simulink model "V605_rotorModel"  (R2025a)
settings: Solver=FixedStepAuto  StartTime=0.0  StopTime=10.0  RelTol=1e-3
undefined symbols (not defined in the file or in its folder): motor
libraries: simulink x1
settings Model: Creator=Ayush_S  LastModifiedBy=Ayush_S

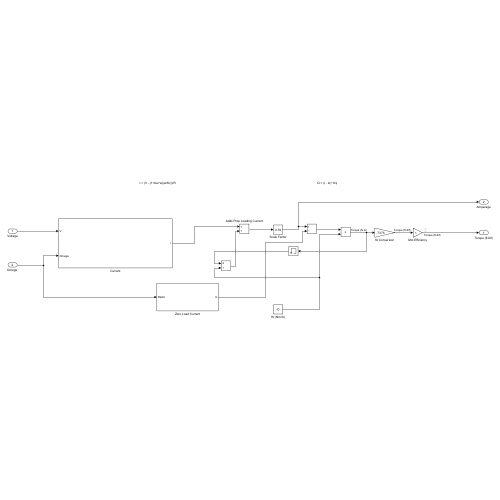
[thumbnail: Simulink's stored preview of the top-level diagram]
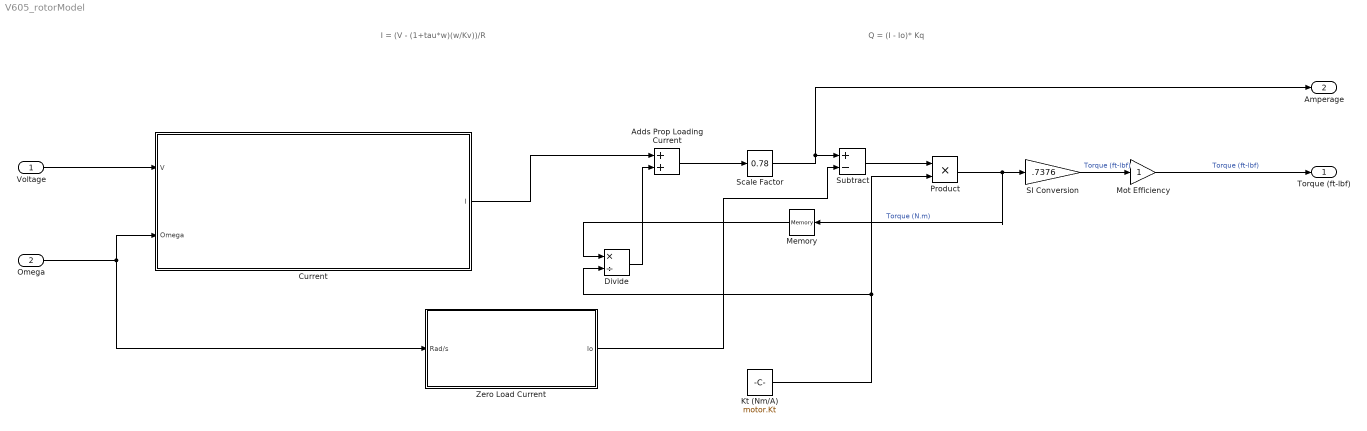
== system V605_rotorModel ==
  note: Q = (I - Io)* Kq
  note: I = (V - (1+tau*w)(w/Kv))/R
  Voltage : Inport
  "Omega " : Inport  Port=2
  Adds Prop Loading Current : Sum
  Current : Subsystem
  Divide : Product  Inputs=*/
  Kt (Nm/A) : Constant  Value=motor.Kt
  Memory : Memory
  Mot Efficiency : Gain
  Product : Product
  SI Conversion : Gain  Gain=.7376
  Scale Factor : simulink/Math Operations/Slider Gain  gain=0.78  low=0  high=2
  Subtract : Sum  Inputs=+-
  Zero Load Current : Subsystem
  Torque (ft-lbf) : Outport
  Amperage : Outport  Port=2
  wires:
  "Omega "/1 -> Current/2(Omega), Zero Load Current/1(Rad/s)
  Zero Load Current/1(Io) -> Subtract/2
  Scale Factor/1 -> Amperage/1, Subtract/1
  Divide/1 -> Adds Prop Loading Current/2
  Product/1 -> Memory/1, SI Conversion/1  "Torque (N.m)"
  Kt (Nm/A)/1 -> Divide/2, Product/2
  Mot Efficiency/1 -> Torque (ft-lbf)/1  "Torque (ft-lbf)"
  Subtract/1 -> Product/1
  Voltage/1 -> Current/1(V)
  Adds Prop Loading Current/1 -> Scale Factor/1
  SI Conversion/1 -> Mot Efficiency/1  "Torque (ft-lbf)"
  Current/1(I) -> Adds Prop Loading Current/1
  Memory/1 -> Divide/1

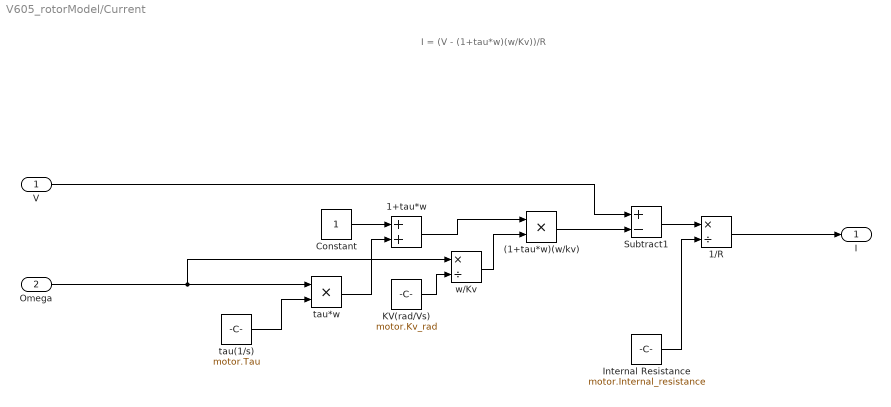
== system V605_rotorModel/Current ==
  note: I = (V - (1+tau*w)(w/Kv))/R
  V : Inport
  Omega : Inport  Port=2
  (1+tau*w)(w/kv) : Product
  1+tau*w : Sum
  1/R : Product  Inputs=*/
  Constant : Constant
  Internal Resistance : Constant  Value=motor.Internal_resistance
  KV(rad/Vs) : Constant  Value=motor.Kv_rad
  Subtract1 : Sum  Inputs=+-
  tau(1/s) : Constant  Value=motor.Tau
  tau*w : Product
  w/Kv : Product  Inputs=*/
  I : Outport
  wires:
  Subtract1/1 -> 1/R/1
  1+tau*w/1 -> (1+tau*w)(w/kv)/1
  (1+tau*w)(w/kv)/1 -> Subtract1/2
  KV(rad/Vs)/1 -> w/Kv/2
  Constant/1 -> 1+tau*w/1
  w/Kv/1 -> (1+tau*w)(w/kv)/2
  tau*w/1 -> 1+tau*w/2
  Internal Resistance/1 -> 1/R/2
  tau(1/s)/1 -> tau*w/2
  V/1 -> Subtract1/1
  Omega/1 -> w/Kv/1, tau*w/1
  1/R/1 -> I/1

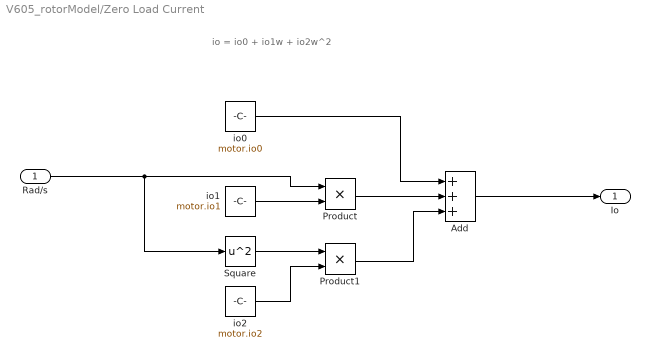
== system V605_rotorModel/Zero Load Current ==
  note: io = io0 + io1w + io2w^2
  Rad/s : Inport
  Add : Sum  Inputs=+++
  Product : Product
  Product1 : Product
  Square : Math  Operator=square
  io0 : Constant  Value=motor.io0
  io1 : Constant  Value=motor.io1
  io2 : Constant  Value=motor.io2
  Io : Outport
  wires:
  io2/1 -> Product1/2
  Square/1 -> Product1/1
  Rad/s/1 -> Product/1, Square/1
  io1/1 -> Product/2
  Add/1 -> Io/1
  Product1/1 -> Add/3
  Product/1 -> Add/2
  io0/1 -> Add/1
